simulink model "superTrame"  (Simulink 8.0)
settings: Solver=ode45  StartTime=0.0  StopTime=10.0  RelTol=1e-3
libraries: simeventsqueue1 x4, simeventsserver1 x4
settings Model: Creator=Nora IZRI  LastModifiedBy=Nora IZRI
settings DataIOCC: SignalLoggingSaveFormat=ModelDataLogs
settings DebuggingCC: FcnCallInpInsideContextMsg=UseLocalSettings
settings GRTTargetCC: CombineOutputUpdateFcns=off  GRTInterface=on
settings SimEventsCC: propDiagAttribOutput=1  propDiagFcnCallOutput=1  propDiagStatOutput=0  propPreventDuplicateEvents=0

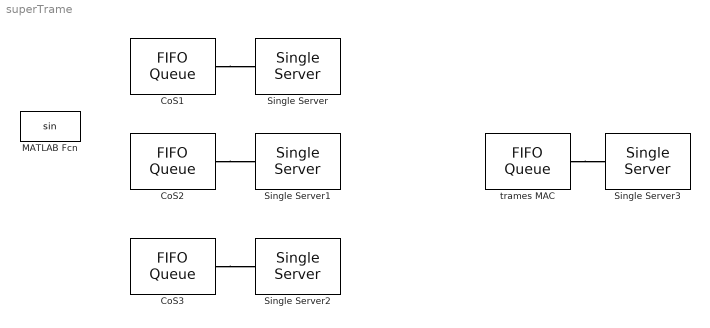
== system superTrame ==
  CoS1 : simeventsqueue1/FIFO Queue  Priority=1  Capacity=25  EnableTOPort=off  StatNumberDeparted=Off  StatNumberInBlock=Off  StatPendingEntity=Off  StatAverageWait=Off  StatAverageQueueLength=Off  StatNumberTimedout=Off
  CoS2 : simeventsqueue1/FIFO Queue  Priority=1  Capacity=25  EnableTOPort=off  StatNumberDeparted=Off  StatNumberInBlock=Off  StatPendingEntity=Off  StatAverageWait=Off  StatAverageQueueLength=Off  StatNumberTimedout=Off
  CoS3 : simeventsqueue1/FIFO Queue  Priority=1  Capacity=25  EnableTOPort=off  StatNumberDeparted=Off  StatNumberInBlock=Off  StatPendingEntity=Off  StatAverageWait=Off  StatAverageQueueLength=Off  StatNumberTimedout=Off
  MATLAB Fcn : MATLABFcn
  Single Server{,1..3} (4 alike) : simeventsserver1/Single Server  Priority=1  ServiceTimeFrom=Dialog  ServiceTime=1  AttributeName=ServiceTime  PriorityServiceCompletion=500  PermitPreemption=off  SortingAttributeName=PriorityAttributeName  SortingDirection=Ascending  WriteToAttribute=off  ResidualAttributeName=ResidualServiceTime  CreateAttribute=on  EnableTOPort=off  StatNumberDeparted=Off  StatNumberInBlock=Off  StatNumberPreempted=Off  StatPendingEntity=Off  StatAverageWait=Off  StatUtilization=Off  StatNumberTimedout=Off
  trames MAC : simeventsqueue1/FIFO Queue  Priority=1  Capacity=25  EnableTOPort=off  StatNumberDeparted=Off  StatNumberInBlock=Off  StatPendingEntity=Off  StatAverageWait=Off  StatAverageQueueLength=Off  StatNumberTimedout=Off
  connections:
  CoS1/RConn1 -- Single Server/LConn1
  CoS2/RConn1 -- Single Server1/LConn1
  CoS3/RConn1 -- Single Server2/LConn1
  trames MAC/RConn1 -- Single Server3/LConn1
